simulink model "Prac1_model"  (R2013b)
settings: Solver=ode45  StartTime=0.0  StopTime=10.0  MaxStep=0.01  RelTol=1e-3
values from neighbouring files (symbols this model uses):
  A = [0, 1; -g/l*cos(theta_0), 0]    [Prac1_setup.m]
  b = [0; 1/(m*l^2)]    [Prac1_setup.m]
  c = [l*cos(theta_0), 0]    [Prac1_setup.m]
  g = 9.81    [Prac1_setup.m]
  l = 1    [Prac1_setup.m]
  m = 1    [Prac1_setup.m]
  theta_0 = asin(u_0/(m*l*g))    [Prac1_setup.m]
  u_0 = 7    [Prac1_setup.m]
  y_0 = l*sin(theta_0)    [Prac1_setup.m]
settings Model: Creator=cvdaalen  LastModifiedBy=cvdaalen

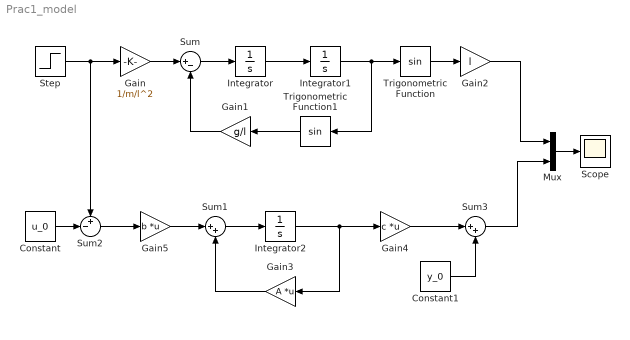
== system Prac1_model ==
  Constant : Constant  Value=u_0
  Constant1 : Constant  Value=y_0
  Gain : Gain  Gain=1/m/l^2
  Gain1 : Gain  Gain=g/l
  Gain2 : Gain  Gain=l
  Gain3 : Gain  Gain=A  Multiplication=Matrix(K*u)
  Gain4 : Gain  Gain=c  Multiplication=Matrix(K*u)
  Gain5 : Gain  Gain=b  Multiplication=Matrix(K*u)
  Integrator : Integrator
  Integrator1 : Integrator  InitialCondition=theta_0
  Integrator2 : Integrator
  Mux : Mux  Inputs=2
  Scope : Scope
  Step : Step  Before=7  After=8  SampleTime=0
  Sum : Sum  Inputs=|+-
  Sum1 : Sum  Inputs=|++
  Sum2 : Sum  Inputs=+-|
  Sum3 : Sum  Inputs=|++
  Trigonometric Function : Trigonometry
  Trigonometric Function1 : Trigonometry
  wires:
  Integrator/1 -> Integrator1/1
  Sum/1 -> Integrator/1
  Gain1/1 -> Sum/2
  Trigonometric Function1/1 -> Gain1/1
  Trigonometric Function/1 -> Gain2/1
  Integrator1/1 -> Trigonometric Function1/1, Trigonometric Function/1
  Gain/1 -> Sum/1
  Step/1 -> Sum2/1, Gain/1
  Sum1/1 -> Integrator2/1
  Gain3/1 -> Sum1/2
  Gain5/1 -> Sum1/1
  Integrator2/1 -> Gain3/1, Gain4/1
  Constant/1 -> Sum2/2
  Sum2/1 -> Gain5/1
  Gain4/1 -> Sum3/1
  Constant1/1 -> Sum3/2
  Mux/1 -> Scope/1
  Gain2/1 -> Mux/1
  Sum3/1 -> Mux/2
